simulink model "MGMinvernadero"  (R2021b)
settings: Solver=ode45  StartTime=0.0  StopTime=168  FixedStep=1  RelTol=1e-3  AbsTol=1e-6
model workspace (MATLAB code in the model file):
  | % load initial conditions and physical properties from file
  | 
  | MGMinvernadero_DATA
values from neighbouring files (symbols this model uses):
  coste_calefac = 0.2809    [MGMinvernadero_DATA.m]
  coste_refrig = -0.2809    [MGMinvernadero_DATA.m]
  cpAire = 1005.4    [MGMinvernadero_DATA.m]
  FlucCalefac = 0.55    [MGMinvernadero_DATA.m]
  FlucRefrig = 0.5    [MGMinvernadero_DATA.m]
  MasaAire = VolInv*1.29    (= 144.48)    [MGMinvernadero_DATA.m]
  MDot = 3000    [MGMinvernadero_DATA.m]
  Qcc = 3600/(1/CoefConvecc+0.06/Ct+1/he)*SInv    (= 1006714.00792)    [MGMinvernadero_DATA.m]
  Req = 0.06/(SInv*CoefConvecc)    (= 3.18066157761e-06)    [MGMinvernadero_DATA.m]
  TempCalefac = 40    [MGMinvernadero_DATA.m]
  TempInt = 20    [MGMinvernadero_DATA.m]
  TempRefrig = 0    [MGMinvernadero_DATA.m]
libraries: simulink x2
Description:
  | Thermal Model of a House
  | 
  | This demo illustrates how you can use Simulink(R) to create the thermal model of
  | a house. This system models the outdoor environment, the thermal
  | characteristics of the house, and the house heating system.
  | 
  | The sldemo_househeat_data.m file initializes data in the model workspace.
  | To make changes, you can edit the model workspace directly or edit the MATLAB(R) file
  | and re-load the model workspace.
  | 
  | To view the model workspace, select View > Model Explorer
  | from the Simulink editor.
  | 
  | Note: Time is given in units of hours
settings Model: Creator=The MathWorks, Inc.  LastModifiedBy=Marta GM
settings SolverCC: AutoScaleAbsTol=off  AlgebraicLoopSolver=TrustRegion
settings DataIOCC: ExternalInput=[]  InitialState=[]  SaveFormat=Array  SaveOutput=off  SaveTime=off  SignalLoggingName=sldemo_househeat_output
settings OptimizationCC: BlockReduction=off  BooleanDataType=off  ExpressionDepthLimit=2147483647  InitFltsAndDblsToZero=on  LifeSpan=inf  BufferReusableBoundary=off
settings DebuggingCC: SaveWithParameterizedLinksMsg=none  UnderspecifiedInitializationDetection=Classic  MergeDetectMultiDrivingBlocksExec=none  SignalResolutionControl=TryResolveAllWithWarning  MultiTaskDSMMsg=warning  MultiTaskCondExecSysMsg=none  IntegerOverflowMsg=none  FcnCallInpInsideContextMsg=warning  BusObjectLabelMismatch=none  StateNameClashWarn=warning  SFUnexpectedBacktrackingDiag=warning  SFNoUnconditionalDefaultTransitionDiag=warning  SFExecutionAtInitializationDiag=none  SFMachineParentedDataDiag=warning  IntegerSaturationMsg=none  ArithmeticOperatorsInVariantConditions=warning
settings HardwareCC: ProdBitPerPointer=32  ProdBitPerSizeT=32  ProdBitPerPtrDiffT=32  ProdLargestAtomicFloat=None  ProdIntDivRoundTo=Undefined  ProdEndianess=Unspecified  ProdWordSize=32  ProdHWDeviceType=32-bit Generic  TargetUnknown=on
settings ModelReferenceCC: PropagateSignalLabelsOutOfModel=off
settings SFSimCC: SimUseLocalCustomCode=off  CustomCodeUndefinedFunction=UseInterfaceOnly
settings RTWCC: RTWUseLocalCustomCode=off
settings CodeAppCC: StateflowObjectComments=on
settings GRTTargetCC: TargetFcnLib=ansi_tfl_tmw.mat  TargetLangStandard=C89/C90 (ANSI)  CombineOutputUpdateFcns=off  GRTInterface=on
settings ConfigComp: CovMetricSettings=dw  CovSaveCumulativeToWorkspaceVar=on  CovSaveSingleToWorkspaceVar=on  CovExternalEMLEnable=off

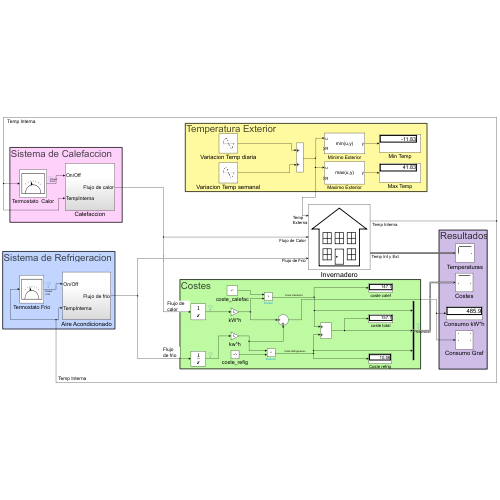
[thumbnail: Simulink's stored preview of the top-level diagram]
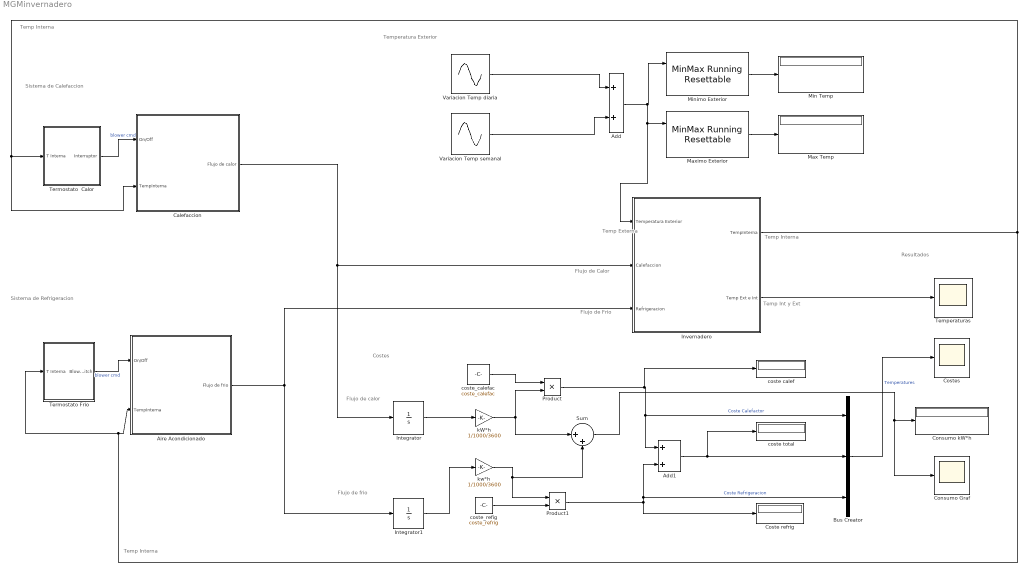
== system MGMinvernadero ==
  note: Flujo de calor
  note: Temp Int y Ext
  note: Temp Interna
  note: Temp Externa
  note: Resultados
  note: Costes
  note: Sistema de Refrigeracion
  note: Sistema de Calefaccion
  note: Temperatura Exterior
  note: Flujo de Calor
  note: Flujo de Frio
  note: Flujo de frio
  note: Temp Interna
  note: Temp Interna
  Add : Sum
  Add1 : Sum
  Aire Acondicionado : Subsystem
  Bus Creator : BusCreator  Inputs=3
  Calefaccion : Subsystem
  Consumo Graf : Scope
  Consumo kW*h : Display
  Coste refrig : Display
  Costes : Scope
  Integrator : Integrator
  Integrator1 : Integrator
  Invernadero : Subsystem
      mask Display: image(fullfile(matlabroot,'toolbox','simulink','simdemos','simgeneral','images','HouseHeatHousePix.svg'))
  Max Temp : Display
  Maximo Exterior : simulink/Math Operations/MinMax Running Resettable  Function=max  vinit=0.0
  Min Temp : Display
  Minimo Exterior : simulink/Math Operations/MinMax Running Resettable  Function=min  vinit=0.0
  Product : Product
  Product1 : Product
  Sum : Sum  Inputs=|++
  Temperaturas : Scope
  Termostato  Calor : Subsystem
      mask Display: image(fullfile(matlabroot,'toolbox','simulink','simdemos','simgeneral','images','HouseHeatThermostatPix.svg'))
  Termostato Frio : Subsystem
      mask Display: image(fullfile(matlabroot,'toolbox','simulink','simdemos','simgeneral','images','HouseHeatThermostatPix.svg'))
  Variacion Temp diaria : Sin  Amplitude=16  Frequency=2*pi/24  SampleTime=0
  Variacion Temp semanal : Sin  Amplitude=12  Bias=15  Frequency=2*pi/168  SampleTime=0
  coste calef : Display
  coste total : Display
  coste_calefac : Constant  Value=coste_calefac
  coste_refig : Constant  Value=coste_refrig
  kW*h : Gain  Gain=1/1000/3600
  kw*h : Gain  Gain=1/1000/3600
  wires:
  Termostato  Calor/1(Interruptor) -> Calefaccion/1(On/Off)  "blower cmd"
  Variacion Temp semanal/1 -> Add/2
  Add/1 -> Minimo Exterior/1, Invernadero/1(Temperatura Exterior), Maximo Exterior/1
  Product/1 -> Add1/1, Bus Creator/1, coste calef/1  "Coste Calefactor"
  Variacion Temp diaria/1 -> Add/1
  Maximo Exterior/1 -> Max Temp/1
  Minimo Exterior/1 -> Min Temp/1
  Termostato Frio/1(Blower switch) -> Aire Acondicionado/1(On/Off)  "blower cmd"
  Aire Acondicionado/1(Flujo de frio) -> Invernadero/3(Refrigeracion), Integrator1/1
  Integrator1/1 -> kw*h/1
  Integrator/1 -> kW*h/1
  Product1/1 -> Add1/2, Bus Creator/3, Coste refrig/1  "Coste Refrigeracion"
  Add1/1 -> coste total/1, Bus Creator/2
  Calefaccion/1(Flujo de calor) -> Invernadero/2("Calefaccion "), Integrator/1
  Invernadero/1(TempInterna) -> Calefaccion/2(TempInterna), Termostato  Calor/1(T Interna), Termostato Frio/1(T Interna), Aire Acondicionado/2(TempInterna)
  Invernadero/2(Temp Ext e Int) -> Temperaturas/1
  Bus Creator/1 -> Costes/1  "Temperatures"
  kw*h/1 -> Sum/2, Product1/1
  coste_calefac/1 -> Product/1
  coste_refig/1 -> Product1/2
  kW*h/1 -> Sum/1, Product/2
  Sum/1 -> Consumo Graf/1, Consumo kW*h/1

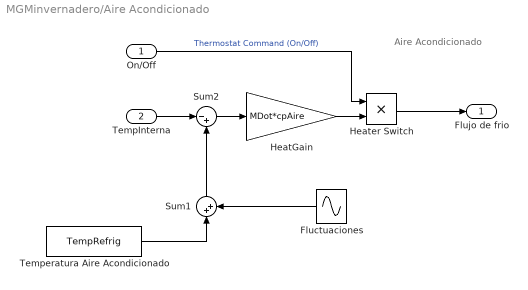
== system MGMinvernadero/Aire Acondicionado ==
  note: Aire Acondicionado
  On/Off : Inport
  TempInterna : Inport  Port=2
  Fluctuaciones : Sin  Amplitude=FlucRefrig  Frequency=1/6  SampleTime=0
  HeatGain : Gain  Gain=MDot*cpAire
  Heater Switch : Product  RndMeth=Zero
  Sum1 : Sum  Inputs=|++
  Sum2 : Sum  Inputs=|-+
  Temperatura Aire Acondicionado : Constant  Value=TempRefrig
  Flujo de frio : Outport  VectorParamsAs1DForOutWhenUnconnected=off
  wires:
  Temperatura Aire Acondicionado/1 -> Sum1/1
  TempInterna/1 -> Sum2/1
  Sum2/1 -> HeatGain/1
  On/Off/1 -> Heater Switch/1  "Thermostat Command (On/Off)"
  HeatGain/1 -> Heater Switch/2
  Heater Switch/1 -> Flujo de frio/1
  Fluctuaciones/1 -> Sum1/2
  Sum1/1 -> Sum2/2

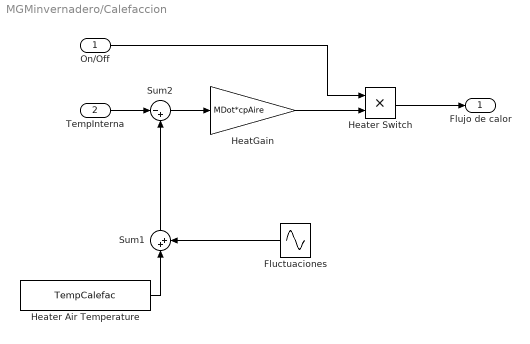
== system MGMinvernadero/Calefaccion ==
  On/Off : Inport
  TempInterna : Inport  Port=2
  Fluctuaciones : Sin  Amplitude=FlucCalefac  Frequency=1/6  SampleTime=0
  HeatGain : Gain  Gain=MDot*cpAire
  Heater Air Temperature : Constant  Value=TempCalefac
  Heater Switch : Product  RndMeth=Zero
  Sum1 : Sum  Inputs=|++
  Sum2 : Sum  Inputs=|-+
  Flujo de calor : Outport  VectorParamsAs1DForOutWhenUnconnected=off
  wires:
  TempInterna/1 -> Sum2/1
  Sum2/1 -> HeatGain/1
  On/Off/1 -> Heater Switch/1
  HeatGain/1 -> Heater Switch/2
  Heater Switch/1 -> Flujo de calor/1
  Heater Air Temperature/1 -> Sum1/1
  Fluctuaciones/1 -> Sum1/2
  Sum1/1 -> Sum2/2

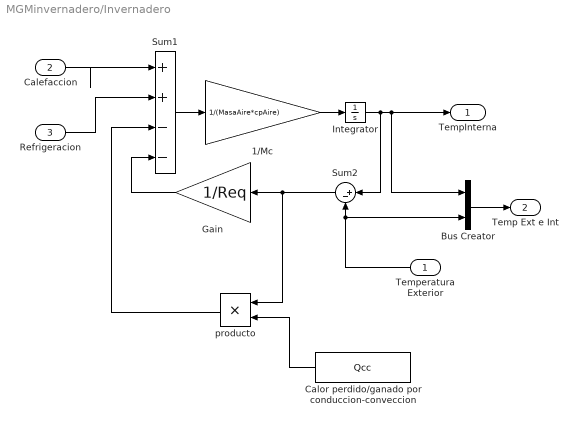
== system MGMinvernadero/Invernadero ==
  Temperatura Exterior : Inport
  "Calefaccion " : Inport  Port=2
  Refrigeracion : Inport  Port=3
  1/Mc : Gain  Gain=1/(MasaAire*cpAire)  SaturateOnIntegerOverflow=on  OutDataTypeStr=Inherit: Same as input  ParamDataTypeStr=Inherit: Same as input
  Bus Creator : BusCreator  Inputs=2
  Calor perdido/ganado por conduccion-conveccion : Constant  Value=Qcc
  Gain : Gain  Gain=1/Req
  Integrator : Integrator  InitialCondition=TempInt
  Sum1 : Sum  Inputs=|++--  InputSameDT=on  SaturateOnIntegerOverflow=on  OutDataTypeStr=Inherit: Same as first input
  Sum2 : Sum  Inputs=|+-  InputSameDT=on  SaturateOnIntegerOverflow=on  OutDataTypeStr=Inherit: Same as first input
  producto : Product  RndMeth=Zero
  TempInterna : Outport  InitialOutput=0  VectorParamsAs1DForOutWhenUnconnected=off
  Temp Ext e Int : Outport  Port=2  InitialOutput=0  VectorParamsAs1DForOutWhenUnconnected=off
  wires:
  Temperatura Exterior/1 -> Sum2/2, Bus Creator/2
  Sum1/1 -> 1/Mc/1
  1/Mc/1 -> Integrator/1
  Integrator/1 -> Sum2/1, Bus Creator/1, TempInterna/1
  Bus Creator/1 -> Temp Ext e Int/1
  Refrigeracion/1 -> Sum1/2
  "Calefaccion "/1 -> Sum1/1
  Gain/1 -> Sum1/4
  Sum2/1 -> producto/1, Gain/1
  producto/1 -> Sum1/3
  Calor perdido/ganado por conduccion-conveccion/1 -> producto/2

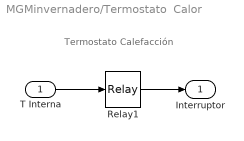
== system MGMinvernadero/Termostato  Calor ==
  note: Termostato Calefacción
  T Interna : Inport
  Relay1 : Relay  OnSwitchValue=23  OffSwitchValue=17  OnOutputValue=0  OffOutputValue=1
  Interruptor : Outport  InitialOutput=0  VectorParamsAs1DForOutWhenUnconnected=off
  wires:
  T Interna/1 -> Relay1/1
  Relay1/1 -> Interruptor/1

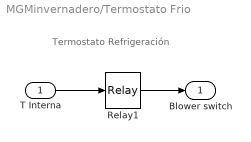
== system MGMinvernadero/Termostato Frio ==
  note: Termostato Refrigeración
  T Interna : Inport
  Relay1 : Relay  OnSwitchValue=35  OffSwitchValue=29
  Blower switch : Outport  InitialOutput=0  VectorParamsAs1DForOutWhenUnconnected=off
  wires:
  T Interna/1 -> Relay1/1
  Relay1/1 -> Blower switch/1
